simulink model "acctest_0422"  (R2021b)
settings: Solver=FixedStepAuto  StartTime=0.0  StopTime=inf  FixedStep=0.01  RelTol=1e-3  EnableMultiTasking=on
libraries: arduinolib x3, simulink x1
settings Model: ExtModeTrigDuration=2  Creator=user  LastModifiedBy=user
settings SolverCC: AutoInsertRateTranBlk=on
settings OptimizationCC: EnhancedBackFolding=on  PassReuseOutputArgsAs=Individual arguments  ZeroExternalMemoryAtStartup=off  ZeroInternalMemoryAtStartup=off  MaxStackSize=64  OptimizeBlockOrder=speed  DifferentSizesBufferReuse=on  OptimizationCustomize=off  EfficientTunableParamExpr=on
settings DebuggingCC: MultiTaskDSMMsg=none  ParameterTunabilityLossMsg=error
settings HardwareCC: ProdBitPerInt=16  ProdBitPerPointer=16  ProdBitPerSizeT=16  ProdBitPerPtrDiffT=16  ProdLargestAtomicFloat=None  ProdWordSize=8  ProdHWDeviceType=Atmel->AVR
settings SFSimCC: MATLABDynamicMemAlloc=off
settings RTWCC: Description=Embedded Coder  SystemTargetFile=ert.tlc  HardwareBoard=Arduino Mega 2560  TemplateMakefile=ert_default_tmf  Toolchain=Arduino AVR  BuildConfiguration=Faster Runs
settings CodeAppCC: ForceParamTrailComments=on  IgnoreCustomStorageClasses=off  OperatorAnnotations=on  SimulinkDataObjDesc=on  SFDataObjDesc=on  InsertBlockDesc=on
settings ERTTargetCC: SupportContinuousTime=on  SupportVariableSizeSignals=on  ExtModeTransport=3  ExtModeStaticAlloc=on  ExtModeStaticAllocSize=2048  ExtModeMexFile=ext_xcp  ExtModeIntrfLevel=Level2 - Open

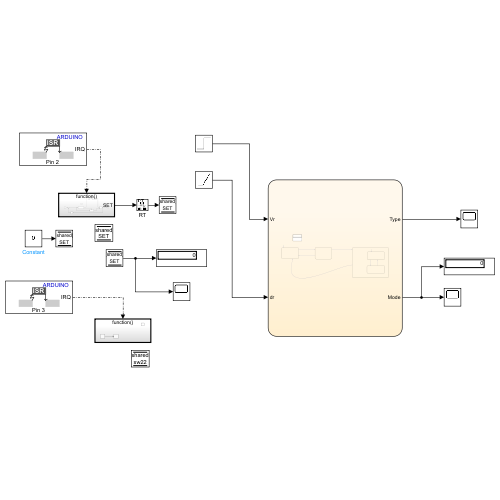
[thumbnail: Simulink's stored preview of the top-level diagram]
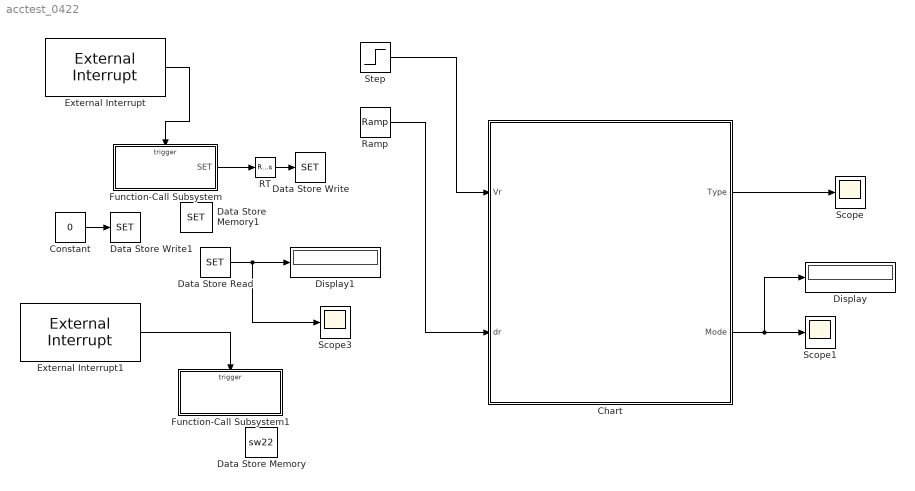
== system acctest_0422 ==
  Chart : Stateflow chart  TreatAsAtomicUnit=on
  Constant : Constant  Value=0  OutDataTypeStr=int8
  Data Store Memory : DataStoreMemory  DataStoreName=sw22  ReadBeforeWriteMsg=warning  WriteAfterWriteMsg=warning  WriteAfterReadMsg=warning  ShareAcrossModelInstances=on  ShowAdditionalParam=off  OutDataTypeStr=int8
  Data Store Memory1 : DataStoreMemory  DataStoreName=SET  ReadBeforeWriteMsg=warning  WriteAfterWriteMsg=warning  WriteAfterReadMsg=warning  ShareAcrossModelInstances=on  ShowAdditionalParam=off  OutDataTypeStr=int8
      settings: LockScale=on
  Data Store Read : DataStoreRead  DataStoreName=SET  IndexOptions=Index vector (dialog)  Indices=1  OutputSizes=1
  Data Store Write : DataStoreWrite  DataStoreName=SET  IndexOptions=Index vector (dialog)  Indices=1  OutputSizes=1
  Data Store Write1 : DataStoreWrite  DataStoreName=SET  IndexOptions=Index vector (dialog)  Indices=1  OutputSizes=1
  Display : Display
  Display1 : Display
  External Interrupt : arduinolib/External Interrupt  Pin=2  PullUp=on  Mode=FALLING  InterruptSimulationInput=off
      settings: SourceProductBaseCode=ARDUINO
  External Interrupt1 : arduinolib/External Interrupt  Pin=3  PullUp=on  Mode=FALLING  InterruptSimulationInput=off
      settings: SourceProductBaseCode=ARDUINO
  Function-Call Subsystem : Subsystem  TreatAsAtomicUnit=on
  Function-Call Subsystem1 : Subsystem  TreatAsAtomicUnit=on
  RT : RateTransition  Deterministic=off  OutPortSampleTime=0.01
  Ramp : simulink/Sources/Ramp  slope=-10  start=0  InitialOutput=500
  Scope : Scope
  Scope1 : Scope
  Scope3 : Scope
  Step : Step  Time=20  Before=-10  After=10  SampleTime=0
  wires:
  Step/1 -> Chart/1(Vr)
  Ramp/1 -> Chart/2(dr)
  Chart/1(Type) -> Scope/1
  Chart/2(Mode) -> Display/1, Scope1/1
  External Interrupt/1 -> Function-Call Subsystem/Trigger
  External Interrupt1/1 -> Function-Call Subsystem1/Trigger
  RT/1 -> Data Store Write/1
  Constant/1 -> Data Store Write1/1
  Data Store Read/1 -> Scope3/1, Display1/1
  Function-Call Subsystem/1(SET) -> RT/1

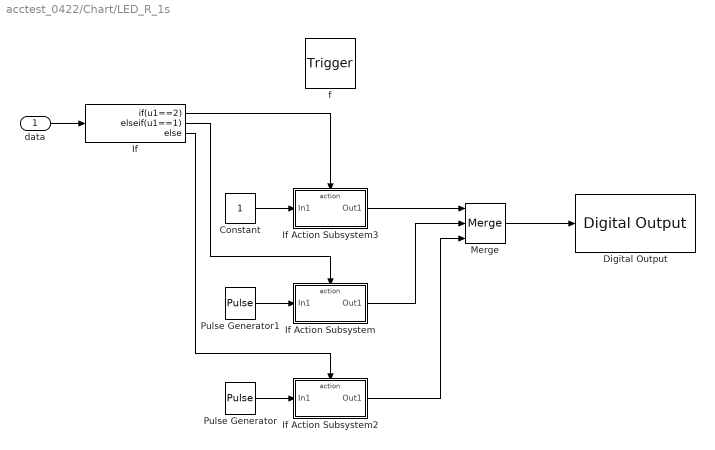
== system acctest_0422/Chart/LED_R_1s ==
  data : Inport  OutDataTypeStr=double  PortDimensions=1
  f : TriggerPort  TriggerType=function-call  VariantControl=(inherit)
      settings: CopyFcn=Stateflow.SLINSF.SimulinkMan.removeBlockPreDeleteFcn  PreDeleteFcn=Stateflow.SLINSF.SimulinkMan.unsafePredeleteFcn
  Constant : Constant
  Digital Output : arduinolib/Digital Output  pinNumber=13  Direction=output  blockPlatform=arduino
  If : If  IfExpression=u1==2  ElseIfExpressions=u1==1
  If Action Subsystem : Subsystem  TreatAsAtomicUnit=on
  If Action Subsystem2 : Subsystem  TreatAsAtomicUnit=on
  If Action Subsystem3 : Subsystem  TreatAsAtomicUnit=on
  Merge : Merge  Inputs=3
  Pulse Generator : DiscretePulseGenerator  Period=200  PulseWidth=100  SampleTime=-1
  Pulse Generator1 : DiscretePulseGenerator  Period=40  PulseWidth=20  SampleTime=-1
  wires:
  data/1 -> If/1
  If/1 -> If Action Subsystem3/Action
  If/2 -> If Action Subsystem/Action
  If/3 -> If Action Subsystem2/Action
  Constant/1 -> If Action Subsystem3/1(In1)
  If Action Subsystem3/1(Out1) -> Merge/1
  Merge/1 -> Digital Output/1
  Pulse Generator1/1 -> If Action Subsystem/1(In1)
  If Action Subsystem/1(Out1) -> Merge/2
  Pulse Generator/1 -> If Action Subsystem2/1(In1)
  If Action Subsystem2/1(Out1) -> Merge/3

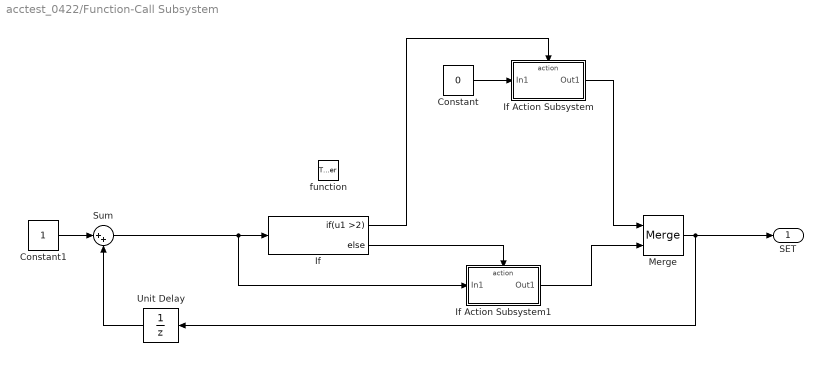
== system acctest_0422/Function-Call Subsystem ==
  function : TriggerPort  TriggerType=function-call  VariantControl=(inherit)
  Constant : Constant  Value=0  OutDataTypeStr=int8
  Constant1 : Constant  OutDataTypeStr=int8
  If : If  IfExpression=u1 >2
  If Action Subsystem : Subsystem  TreatAsAtomicUnit=on
  If Action Subsystem1 : Subsystem  TreatAsAtomicUnit=on
  Merge : Merge
  Sum : Sum  Inputs=|++
  Unit Delay : UnitDelay  SampleTime=-1  HasFrameUpgradeWarning=on
  SET : Outport
  wires:
  If Action Subsystem/1(Out1) -> Merge/1
  Constant/1 -> If Action Subsystem/1(In1)
  Sum/1 -> If Action Subsystem1/1(In1), If/1
  Unit Delay/1 -> Sum/2
  Merge/1 -> Unit Delay/1, SET/1
  If/1 -> If Action Subsystem/Action
  If/2 -> If Action Subsystem1/Action
  If Action Subsystem1/1(Out1) -> Merge/2
  Constant1/1 -> Sum/1

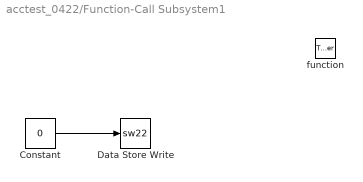
== system acctest_0422/Function-Call Subsystem1 ==
  function : TriggerPort  TriggerType=function-call  VariantControl=(inherit)
  Constant : Constant  Value=0  OutDataTypeStr=int8
  Data Store Write : DataStoreWrite  DataStoreName=sw22  IndexOptions=Index vector (dialog)  Indices=1  OutputSizes=1
  wires:
  Constant/1 -> Data Store Write/1

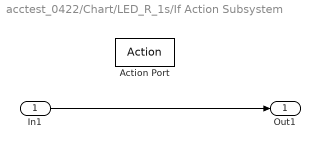
== system acctest_0422/Chart/LED_R_1s/If Action Subsystem ==
  In1 : Inport
  Action Port : ActionPort  ActionPortLabel=elseif(u1==1)
  Out1 : Outport
  wires:
  In1/1 -> Out1/1

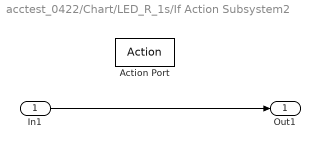
== system acctest_0422/Chart/LED_R_1s/If Action Subsystem2 ==
  In1 : Inport
  Action Port : ActionPort  ActionPortLabel=else
  Out1 : Outport
  wires:
  In1/1 -> Out1/1

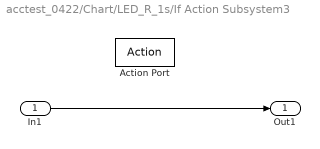
== system acctest_0422/Chart/LED_R_1s/If Action Subsystem3 ==
  In1 : Inport
  Action Port : ActionPort  ActionPortLabel=if(u1==2)
  Out1 : Outport
  wires:
  In1/1 -> Out1/1

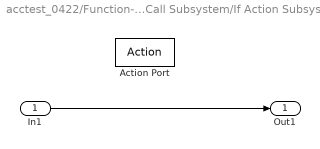
== system acctest_0422/Function-Call Subsystem/If Action Subsystem ==
  In1 : Inport
  Action Port : ActionPort  ActionPortLabel=if(u1 >2)
  Out1 : Outport
  wires:
  In1/1 -> Out1/1

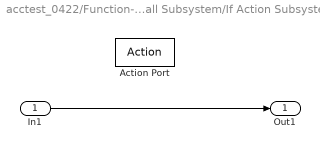
== system acctest_0422/Function-Call Subsystem/If Action Subsystem1 ==
  In1 : Inport
  Action Port : ActionPort  ActionPortLabel=else
  Out1 : Outport
  wires:
  In1/1 -> Out1/1

== stateflow chart acctest_0422/Chart ==
  state LED_R_1s(data) [function]
  state ACC_standby
    Mode=1;
    LED_R_1s(1);
  state ACC_off
    Mode=0;
    sw22=1;
    SET=0;
    LED_R_1s(0);
  state ACC_active
    Mode=2;
    LED_R_1s(2);
    state Speed_control
      Type=0;
    state Timegap_control
      Type=1;
    (default) -> Speed_control
    Speed_control -> Timegap_control : [dr<200&&Vr>0]
    Timegap_control -> Speed_control : [dr>200||Vr<0]
  (default) -> ACC_off
  ACC_standby -> ACC_active [order 1] : [SET==2]
  ACC_off -> ACC_standby : [SET==1]
  ACC_standby -> ACC_off [order 2] : [sw22==0]
  ACC_active -> ACC_off : [SET==0||sw22==0]
  data: data function_input double size=1; Vr input; dr input; Type output; Mode output; sw22 data_store_memory; SET data_store_memory
